simulink model "Moisture_Control"  (R2023b)
settings: Solver=FixedStepDiscrete  StartTime=0.0  StopTime=10000  FixedStep=1e-3  MaxStep=1e-3  RelTol=1e-3  EnableMultiTasking=on
settings Model: NumberOfSteps=200000  Creator=gaafa  LastModifiedBy=gaafa
settings SolverCC: AutoInsertRateTranBlk=on
settings OptimizationCC: DefaultParameterBehavior=Inlined  UseDivisionForNetSlopeComputation=on  GainParamInheritBuiltInType=on  UseFloatMulNetSlope=on  InlineInvariantSignals=on  PassReuseOutputArgsAs=Individual arguments  ZeroExternalMemoryAtStartup=off  ZeroInternalMemoryAtStartup=off  NoFixptDivByZeroProtection=on  EfficientFloat2IntCast=on  LifeSpan=1  OptimizeBlockOrder=speed  DifferentSizesBufferReuse=on  EfficientTunableParamExpr=on
settings DebuggingCC: ParameterTunabilityLossMsg=error
settings HardwareCC: ProdBitPerPointer=32  ProdBitPerSizeT=32  ProdBitPerPtrDiffT=32  ProdLargestAtomicFloat=None  ProdWordSize=32  ProdLongLongMode=on  ProdHWDeviceType=Atmel->AVR (32-bit)
settings SFSimCC: MATLABDynamicMemAlloc=off
settings RTWCC: Description=Embedded Coder  SystemTargetFile=ert.tlc  TemplateMakefile=ert_default_tmf
settings CodeAppCC: ForceParamTrailComments=on  IgnoreCustomStorageClasses=off  OperatorAnnotations=on  SimulinkDataObjDesc=on  SFDataObjDesc=on  CustomSymbolStrGlobalVar=rt$N$M  CustomSymbolStrType=$N$M  CustomSymbolStrFcn=$N$M$F  CustomSymbolStrMacro=$N$M  InsertBlockDesc=on
settings ERTTargetCC: TargetLangStandard=C99 (ISO)  GenerateSampleERTMain=on  IncludeMdlTerminateFcn=off  CombineSignalStateStructs=on  SuppressErrorStatus=on  SupportAbsoluteTime=off  SupportComplex=off  InlinedParameterPlacement=NonHierarchical  ERTCustomFileTemplate=example_file_process.tlc  ERTFilePackagingFormat=CompactWithDataFile

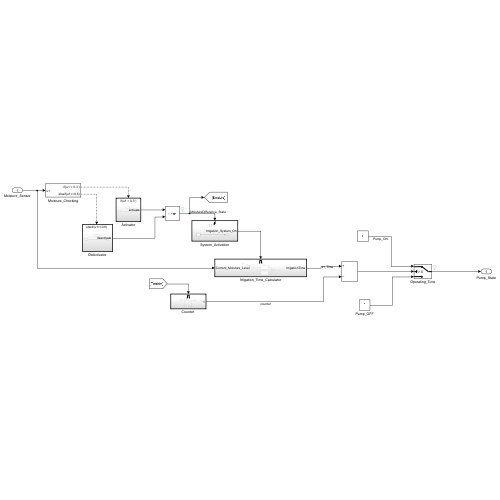
[thumbnail: Simulink's stored preview of the top-level diagram]
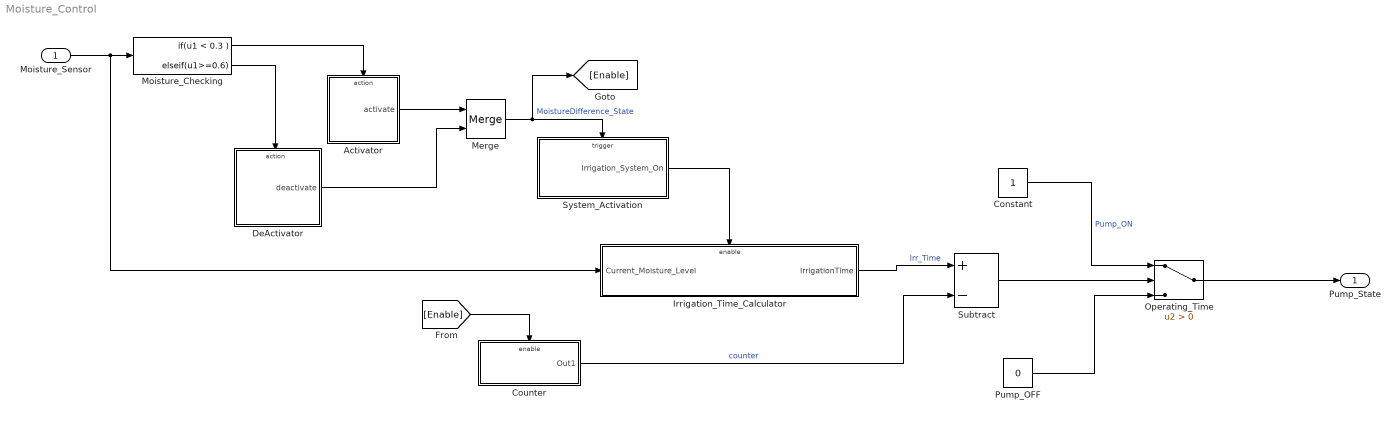
== system Moisture_Control ==
  Moisture_Sensor : Inport
  Activator : Subsystem  TreatAsAtomicUnit=on
  Constant : Constant
  "Counter " : Subsystem
  DeActivator : Subsystem  TreatAsAtomicUnit=on
  Irrigation_Time_Calculator : Subsystem  TreatAsAtomicUnit=on
  Merge : Merge
  Moisture_Checking : If  IfExpression=u1 < 0.3  ElseIfExpressions=u1>=0.6  ShowElse=off
  Operating_Time : Switch  Criteria=u2 > Threshold  SaturateOnIntegerOverflow=off  InputSameDT=off
  Pump_OFF : Constant  Value=0
  Subtract : Sum  Inputs=+-
  System_Activation : Subsystem  TreatAsAtomicUnit=on
  Pump_State : Outport
  wires:
  Moisture_Checking/1 -> Activator/Action
  Moisture_Checking/2 -> DeActivator/Action
  Activator/1(activate) -> Merge/1
  DeActivator/1(deactivate) -> Merge/2
  System_Activation/1(Irrigation_System_On) -> Irrigation_Time_Calculator/Enable
  Moisture_Sensor/1 -> Moisture_Checking/1, Irrigation_Time_Calculator/1(Current_Moisture_Level)
  Constant/1 -> Operating_Time/1  "Pump_ON"
  Pump_OFF/1 -> Operating_Time/3
  Operating_Time/1 -> Pump_State/1
  Irrigation_Time_Calculator/1(IrrigationTime) -> Subtract/1  "Irr_Time"
  "Counter "/1(Out1) -> Subtract/2  "counter"
  Merge/1 -> [Enable], System_Activation/Trigger  "MoistureDifference_State"
  Subtract/1 -> Operating_Time/2
  [Enable] -> "Counter "/Enable

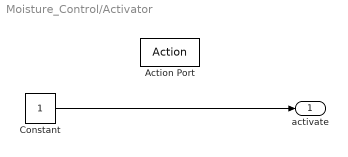
== system Moisture_Control/Activator ==
  Action Port : ActionPort  InitializeStates=reset  ActionPortLabel=if(u1 < 0.3 )
  Constant : Constant
  activate : Outport
  wires:
  Constant/1 -> activate/1

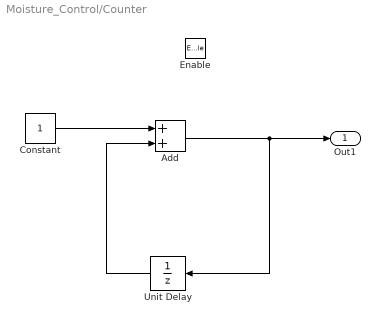
== system Moisture_Control/Counter  ==
  Enable : EnablePort  StatesWhenEnabling=reset
  Add : Sum
  Constant : Constant
  Unit Delay : UnitDelay  HasFrameUpgradeWarning=on
  Out1 : Outport
  wires:
  Constant/1 -> Add/1
  Unit Delay/1 -> Add/2
  Add/1 -> Unit Delay/1, Out1/1

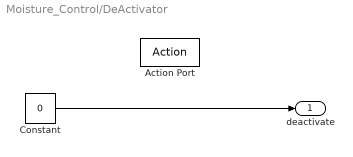
== system Moisture_Control/DeActivator ==
  Action Port : ActionPort  ActionPortLabel=elseif(u1>=0.6)
  Constant : Constant  Value=0
  deactivate : Outport
  wires:
  Constant/1 -> deactivate/1

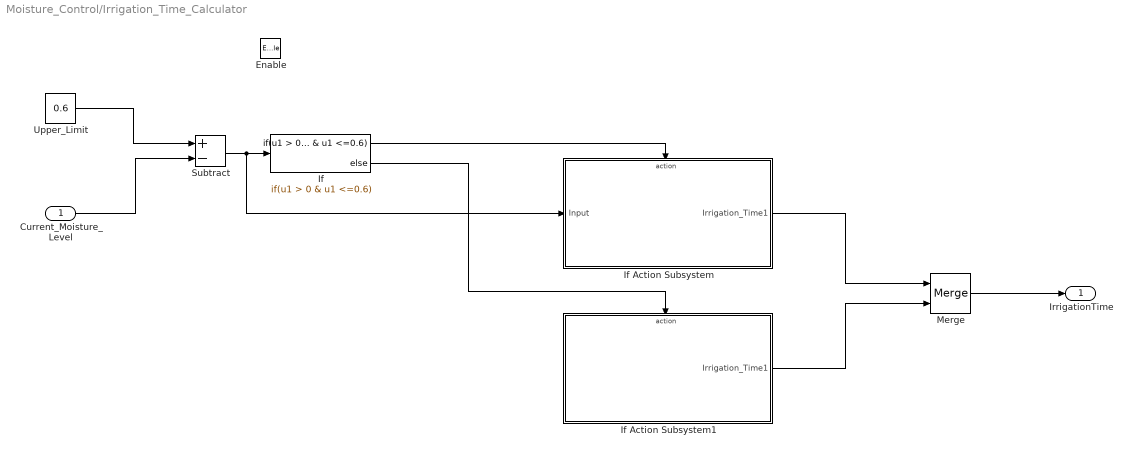
== system Moisture_Control/Irrigation_Time_Calculator ==
  Current_Moisture_Level : Inport
  Enable : EnablePort  StatesWhenEnabling=reset
  If : If  IfExpression=u1 > 0 & u1 <=0.6
  If Action Subsystem : Subsystem  TreatAsAtomicUnit=on
  If Action Subsystem1 : Subsystem  TreatAsAtomicUnit=on
  Merge : Merge
  Subtract : Sum  Inputs=+-
  Upper_Limit : Constant  Value=0.6
  IrrigationTime : Outport
  wires:
  Upper_Limit/1 -> Subtract/1
  Current_Moisture_Level/1 -> Subtract/2
  Subtract/1 -> If Action Subsystem/1(Input), If/1
  If/1 -> If Action Subsystem/Action
  If/2 -> If Action Subsystem1/Action
  If Action Subsystem/1(Irrigation_Time1) -> Merge/1
  If Action Subsystem1/1(Irrigation_Time1) -> Merge/2
  Merge/1 -> IrrigationTime/1

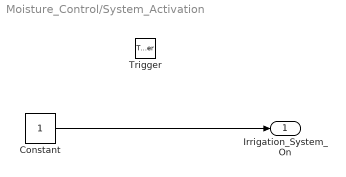
== system Moisture_Control/System_Activation ==
  Trigger : TriggerPort  VariantControl=(inherit)
  Constant : Constant
  Irrigation_System_On : Outport
  wires:
  Constant/1 -> Irrigation_System_On/1

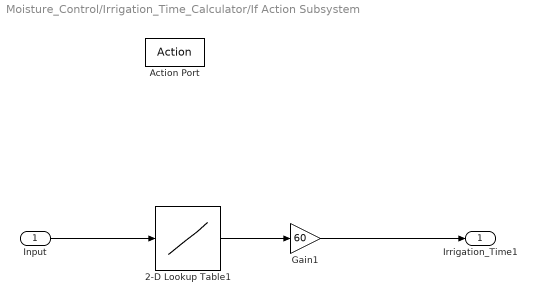
== system Moisture_Control/Irrigation_Time_Calculator/If Action Subsystem ==
  Input : Inport
  Action Port : ActionPort  ActionPortLabel=if(u1 > 0 & u1 <=0.6)
  2-D Lookup Table1 : Lookup_n-D  NumberOfTableDimensions=1  BreakpointsForDimension1=[0 0.1 0.2 0.3 0.4 0.5 0.6]  BreakpointsForDimension2=[1:3]  Table=[0 5 10 15 20 25 30]  InternalRulePriority=Speed  RndMeth=Simplest
  Gain1 : Gain  Gain=60
  Irrigation_Time1 : Outport
  wires:
  2-D Lookup Table1/1 -> Gain1/1
  Gain1/1 -> Irrigation_Time1/1
  Input/1 -> 2-D Lookup Table1/1

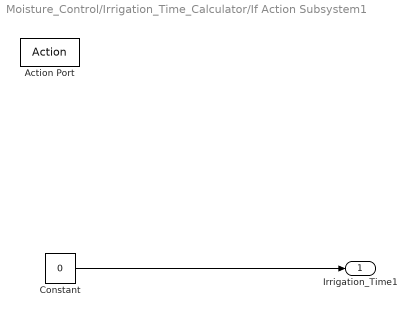
== system Moisture_Control/Irrigation_Time_Calculator/If Action Subsystem1 ==
  Action Port : ActionPort  ActionPortLabel=else
  Constant : Constant  Value=0
  Irrigation_Time1 : Outport
  wires:
  Constant/1 -> Irrigation_Time1/1
